simulink model "Russia_EU_Ukraine_gas_pipeline"  (R2021a)
settings: Solver=ode45  StartTime=0.0  StopTime=100  RelTol=1e-3  EnableMultiTasking=on
undefined symbols (not defined in the file): Tab, Tba, Tca, Tcb
settings Model: Creator=Luan Nguyen  LastModifiedBy=fmendoz2
settings SolverCC: AlgebraicLoopSolver=TrustRegion
settings DataIOCC: LimitDataPoints=on  SaveFormat=Array  SignalLoggingSaveFormat=ModelDataLogs  ReturnWorkspaceOutputs=off
settings OptimizationCC: ExpressionDepthLimit=2147483647  LifeSpan=inf
settings DebuggingCC: UnderspecifiedInitializationDetection=Classic  MergeDetectMultiDrivingBlocksExec=none  IgnoredZcDiagnostic=none  MultiTaskDSMMsg=warning  MultiTaskCondExecSysMsg=none  StateNameClashWarn=warning  SFUnexpectedBacktrackingDiag=warning  SFNoUnconditionalDefaultTransitionDiag=warning  SFExecutionAtInitializationDiag=none  SFMachineParentedDataDiag=warning  ArithmeticOperatorsInVariantConditions=warning
settings HardwareCC: ProdBitPerPointer=32  ProdBitPerSizeT=32  ProdBitPerPtrDiffT=32  ProdLargestAtomicFloat=None  ProdIntDivRoundTo=Undefined  ProdEndianess=Unspecified  ProdWordSize=32  ProdHWDeviceType=32-bit Generic
settings ModelReferenceCC: PropagateSignalLabelsOutOfModel=off
settings SFSimCC: SimUseLocalCustomCode=off  CustomCodeUndefinedFunction=UseInterfaceOnly
settings RTWCC: RTWUseLocalCustomCode=off
settings CodeAppCC: StateflowObjectComments=on
settings GRTTargetCC: TargetLangStandard=C89/C90 (ANSI)
settings ConfigComp: CovMetricSettings=dw  CovSaveCumulativeToWorkspaceVar=on  CovSaveSingleToWorkspaceVar=on  CovExternalEMLEnable=off  CovSFcnEnable=off

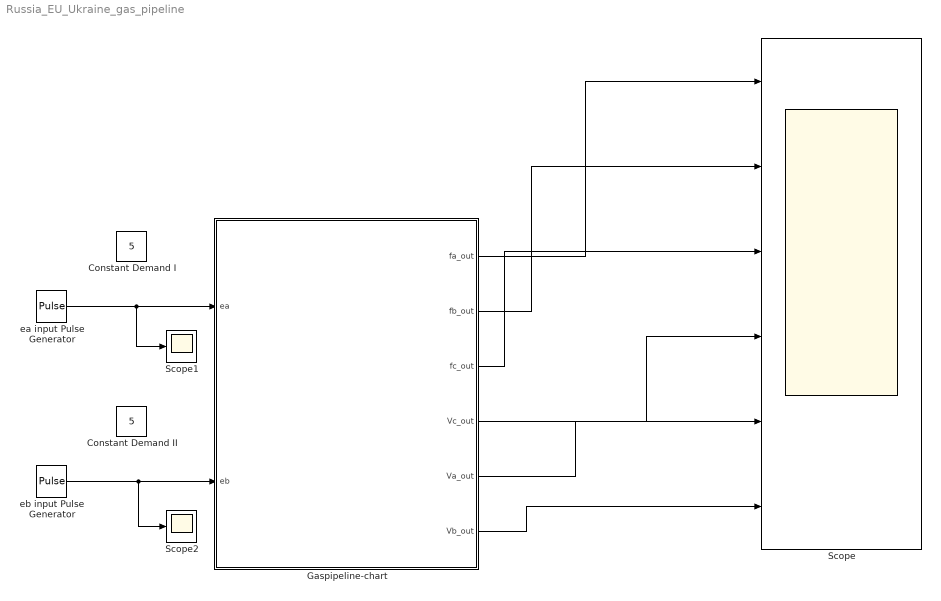
== system Russia_EU_Ukraine_gas_pipeline ==
  Constant Demand I : Constant  Value=5
  Constant Demand II : Constant  Value=5
  Gaspipeline-chart : Stateflow chart  TreatAsAtomicUnit=on
  Scope : Scope  NumInputPorts=6
  Scope1 : Scope
  Scope2 : Scope
  ea input Pulse Generator : DiscretePulseGenerator  PulseType=Time based  Amplitude=5  Period=10
  eb input Pulse Generator : DiscretePulseGenerator  PulseType=Time based  Amplitude=-5  Period=10
  wires:
  Gaspipeline-chart/1(fa_out) -> Scope/1
  Gaspipeline-chart/2(fb_out) -> Scope/2
  Gaspipeline-chart/3(fc_out) -> Scope/3
  Gaspipeline-chart/4(Vc_out) -> Scope/4
  Gaspipeline-chart/5(Va_out) -> Scope/5
  Gaspipeline-chart/6(Vb_out) -> Scope/6
  ea input Pulse Generator/1 -> Gaspipeline-chart/1(ea), Scope1/1
  eb input Pulse Generator/1 -> Gaspipeline-chart/2(eb), Scope2/1

== stateflow chart Russia_EU_Ukraine_gas_pipeline/Gaspipeline-chart ==
  settings: updateMethod=CONTINUOUS
  state PlantModel [parallel]
    settings: executionOrder=4
    state Plant
      du:
      Va_dot = fa; Va_out = Va; fa_dot = 0; fa_out = fa;
      Vb_dot = fb; Vb_out = Vb; fb_dot = 0; fb_out = fb;
      Vc_dot = fc; Vc_out = Vc; fc_dot = 0; fc_out = fc;
  state C_controller_RUSSIA [parallel]
    settings: executionOrder=3
    state C2
      du:
      zc_dot = 1;
    state C1
    (default) -> C1 : {zc = 0; tmpC = 0;}
    C2 -> C1 : [zc >=1]
        | {fc = fc+tmpC; zc = 0;}
    C1 -> C2 : [ea +eb >0 || ea + eb <0]
        | {tmpC = ea+eb;}
  state B_controller_UKRAINE [parallel]
    settings: executionOrder=1
    state ModeB3
      du:
      zb_dot = 1;
    state ModeB5
      du:
      zb_dot = 1;
    state ModeB1
    state ModeB4
      du:
      zb_dot = 1;
    (default) -> ModeB1 : {fb = 5; fc = 10; fa = 5; zb = 0; tmpB = 0;}
    ModeB5 -> ModeB1 : [zb >= 1]
        | {fb = fb+ tmpB;zb = 0;}
    ModeB3 -> ModeB1 : [zb >= Tba]
        | {fb = fb+tmpB; zb = 0;}
    ModeB1 -> ModeB3 [order 2] : [eb > 0 && eb+ea <= 0]{tmpB = eb;}
    ModeB1 -> ModeB5 [order 3] : [eb <= 0 ]
        | {tmpB = eb;}
    ModeB4 -> ModeB1 : [zb >= Tcb && eb+ea > 0]
        | {fb = fb+tmpB; zb = 0;}
    ModeB1 -> ModeB4 [order 1] : [eb > 0 && eb+ea > 0]{tmpB = eb;}
  state A_controller_EU [parallel]
    settings: executionOrder=2
    state ModeA3
      du:
      za_dot = 1;
    state ModeA5
      du:
      za_dot = 1;
    state ModeA1
      du:
    state ModeA4
      du:
      za_dot = 1;
    (default) -> ModeA1 : {za = 0;tmpA = 0;}
    ModeA5 -> ModeA1 : [za >= 1]
        | {fa = fa+ tmpA;za = 0;}
    ModeA3 -> ModeA1 : [za >= Tba]
        | {fa = fa+tmpA; za = 0;}
    ModeA1 -> ModeA5 [order 3] : [ea <= 0 ]
        | {tmpA = ea;}
    ModeA1 -> ModeA3 [order 1] : [ea > 0&&eb+ea <= 0]{tmpA = ea;}
    ModeA4 -> ModeA1 : [za >= Tca]
        | {fa = fa+tmpA; za = 0;}
    ModeA1 -> ModeA4 [order 2] : [ea > 0&&eb+ea > 0]{tmpA = ea;}
  data: za local double; zb local double; fa local double; fa_out output double; ea input double; fb local double; fb_out output double; fc local double; fc_out output double; Va local double; Vb local double; Vc local double; Vc_out output double; Va_out output double; Vb_out output double; Tba parameter double; Tca parameter double; Tcb parameter double; eb input double; Tab parameter double; zc local double; tmpA local double; tmpB local double; tmpC local double
  data za settings: updateMethod=SF_CONTINUOUS_TIME_DATA
  data zb settings: updateMethod=SF_CONTINUOUS_TIME_DATA
  data fa settings: updateMethod=SF_CONTINUOUS_TIME_DATA
  data fb settings: updateMethod=SF_CONTINUOUS_TIME_DATA
  data fc settings: updateMethod=SF_CONTINUOUS_TIME_DATA
  data Va settings: updateMethod=SF_CONTINUOUS_TIME_DATA
  data Vb settings: updateMethod=SF_CONTINUOUS_TIME_DATA
  data Vc settings: updateMethod=SF_CONTINUOUS_TIME_DATA
  data zc settings: updateMethod=SF_CONTINUOUS_TIME_DATA
